simulink library "disturbance_lib"  (R2018b)
settings: Solver=VariableStepAuto  StartTime=0.0  StopTime=10.0  RelTol=1e-3
libraries: simulink x1
settings Model: Creator=sebbe  LastModifiedBy=sebbe

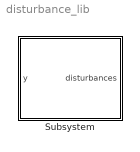
== system disturbance_lib ==
  Subsystem : Subsystem

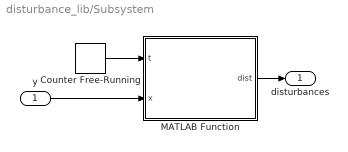
== system disturbance_lib/Subsystem ==
  y : Inport
  Counter Free-Running : simulink/Sources/Counter Free-Running  NumBits=32  tsamp=continuous_h
  MATLAB Function : MATLAB Function  TreatAsAtomicUnit=on
  disturbances : Outport
  wires:
  y/1 -> MATLAB Function/2(x)
  Counter Free-Running/1 -> MATLAB Function/1(t)
  MATLAB Function/1(dist) -> disturbances/1

== matlab function disturbance_lib/Subsystem/MATLAB Function ==
  data: dist output; t input; x input; disturbances parameter
function dist = calc_disturbances(t, x, disturbances)
% Disturbances is 4-C-X matrix of C points in X steps
% First dimension is position x, y, z and magnitude M
% Output dist is 4-C-N matrix of [x;y;z;dist] for C disturbances on N drones
i = t+1; % Current time index
[~, C, ~] = size(disturbances);
[~, N] = size(x);
if i > numel(disturbances(1,1,:))
    i = uint32(1);
end
dist = zeros(4, C, N);
for n=1:N
    for c=1:C
        dist(1:3,c,n) = x(1:3,n) - disturbances(1:3,c,i);
        dist(4,c,n) = norm(dist(1:3,c,n));
        dist(1:3,c,n) = dist(1:3,c,n)*disturbances(4,c,i)/dist(4,c,n);
    end
end
